simulink model "sistema2ordem"  (Simulink 7.9)
settings: Solver=ode45  StartTime=0.0  StopTime=10.0  RelTol=1e-3
settings Model: Creator=Hugo  LastModifiedBy=Hugo
settings DataIOCC: LimitDataPoints=off

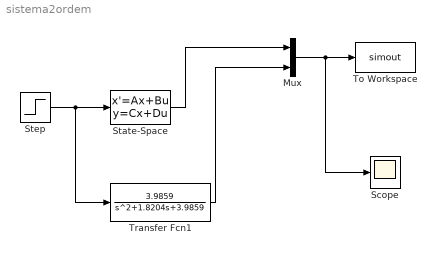
== system sistema2ordem ==
  Mux : Mux  Inputs=2
  Scope : Scope
      settings: SampleInput=on  SampleTime=0.01
  State-Space : StateSpace  A=[-1.824 -2 ; 2 0]  B=[2 ; 0]  C=[0 1]  D=0
  Step : Step  Time=0  After=2  SampleTime=0
  To Workspace : ToWorkspace  VariableName=simout  SampleTime=-1
  Transfer Fcn1 : TransferFcn  Numerator=[3.9859]  Denominator=[1 1.8204 3.9859]
  wires:
  Step/1 -> Transfer Fcn1/1, State-Space/1
  Mux/1 -> To Workspace/1, Scope/1
  Transfer Fcn1/1 -> Mux/2
  State-Space/1 -> Mux/1
